simulink model "Distribution"  (R2018b)
settings: Solver=ode45  StartTime=0.0  StopTime=100  RelTol=1e-3
libraries: simeventslib x20
(part 1 of 2)
settings Model: Creator=tsprock3  LastModifiedBy=tas5
settings DataIOCC: LimitDataPoints=on  SaveFormat=Array
settings OptimizationCC: BlockReduction=off  BooleanDataType=off  LifeSpan=inf
settings DebuggingCC: SaveWithParameterizedLinksMsg=none  UnderspecifiedInitializationDetection=Classic  MergeDetectMultiDrivingBlocksExec=none  SignalResolutionControl=TryResolveAllWithWarning  AllowSymbolicDim=off  SFUnexpectedBacktrackingDiag=warning  SFNoUnconditionalDefaultTransitionDiag=warning  SFExecutionAtInitializationDiag=none
settings HardwareCC: ProdBitPerPointer=32  ProdBitPerSizeT=32  ProdBitPerPtrDiffT=32  ProdLargestAtomicFloat=None  ProdIntDivRoundTo=Undefined  ProdEndianess=Unspecified  ProdWordSize=32  ProdHWDeviceType=32-bit Generic  TargetUnknown=on
settings ModelReferenceCC: PropagateSignalLabelsOutOfModel=off
settings SFSimCC: SimUseLocalCustomCode=off
settings RTWCC: RTWUseLocalCustomCode=off
settings CodeAppCC: StateflowObjectComments=on
settings GRTTargetCC: TargetLangStandard=C89/C90 (ANSI)  GeneratePreprocessorConditionals=Disable all
settings ConfigComp: CovMetricSettings=dw  CovHtmlReporting=on  CovSaveCumulativeToWorkspaceVar=on  CovSaveSingleToWorkspaceVar=on  CovExternalEMLEnable=off
settings SimEventsCC: propMaxDesBlkSimulEvents=100000  propMaxDesMdlSimulEvents=1000000

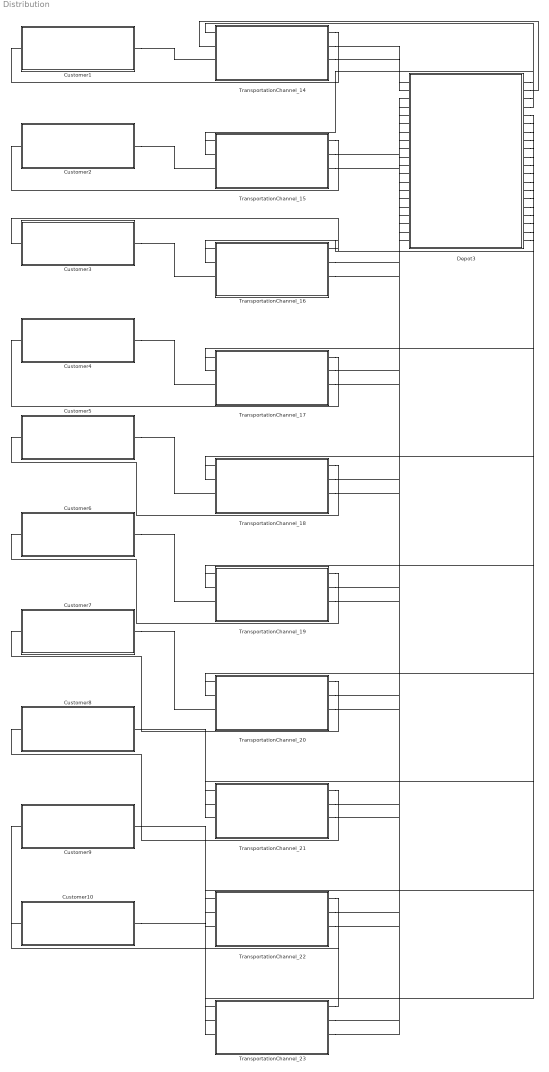
== system Distribution ==
  Customer1 : Subsystem
  Customer10 : Subsystem
  Customer2 : Subsystem
  Customer3 : Subsystem
  Customer4 : Subsystem
  Customer5 : Subsystem
  Customer6 : Subsystem
  Customer7 : Subsystem
  Customer8 : Subsystem
  Customer9 : Subsystem
  Depot3 : Subsystem
  TransportationChannel_14 : Subsystem
  TransportationChannel_15 : Subsystem
  TransportationChannel_16 : Subsystem
  TransportationChannel_17 : Subsystem
  TransportationChannel_18 : Subsystem
  TransportationChannel_19 : Subsystem
  TransportationChannel_20 : Subsystem
  TransportationChannel_21 : Subsystem
  TransportationChannel_22 : Subsystem
  TransportationChannel_23 : Subsystem
  connections:
  Depot3/RConn1 -- TransportationChannel_14/LConn1
  TransportationChannel_14/RConn1 -- Customer1/LConn1
  Depot3/RConn2 -- TransportationChannel_14/LConn2
  TransportationChannel_14/RConn2 -- Depot3/LConn1
  Customer1/RConn1 -- TransportationChannel_14/LConn3
  TransportationChannel_14/RConn3 -- Depot3/LConn2
  Depot3/RConn3 -- TransportationChannel_15/LConn1
  TransportationChannel_15/RConn1 -- Customer2/LConn1
  Depot3/RConn4 -- TransportationChannel_15/LConn2
  TransportationChannel_15/RConn2 -- Depot3/LConn3
  Customer2/RConn1 -- TransportationChannel_15/LConn3
  TransportationChannel_15/RConn3 -- Depot3/LConn4
  Depot3/RConn5 -- TransportationChannel_16/LConn1
  TransportationChannel_16/RConn1 -- Customer3/LConn1
  Depot3/RConn6 -- TransportationChannel_16/LConn2
  TransportationChannel_16/RConn2 -- Depot3/LConn5
  Customer3/RConn1 -- TransportationChannel_16/LConn3
  TransportationChannel_16/RConn3 -- Depot3/LConn6
  Depot3/RConn7 -- TransportationChannel_17/LConn1
  TransportationChannel_17/RConn1 -- Customer4/LConn1
  Depot3/RConn8 -- TransportationChannel_17/LConn2
  TransportationChannel_17/RConn2 -- Depot3/LConn7
  Customer4/RConn1 -- TransportationChannel_17/LConn3
  TransportationChannel_17/RConn3 -- Depot3/LConn8
  Depot3/RConn9 -- TransportationChannel_18/LConn1
  TransportationChannel_18/RConn1 -- Customer5/LConn1
  Depot3/RConn10 -- TransportationChannel_18/LConn2
  TransportationChannel_18/RConn2 -- Depot3/LConn9
  Customer5/RConn1 -- TransportationChannel_18/LConn3
  TransportationChannel_18/RConn3 -- Depot3/LConn10
  Depot3/RConn11 -- TransportationChannel_19/LConn1
  TransportationChannel_19/RConn1 -- Customer6/LConn1
  Depot3/RConn12 -- TransportationChannel_19/LConn2
  TransportationChannel_19/RConn2 -- Depot3/LConn11
  Customer6/RConn1 -- TransportationChannel_19/LConn3
  TransportationChannel_19/RConn3 -- Depot3/LConn12
  Depot3/RConn13 -- TransportationChannel_20/LConn1
  TransportationChannel_20/RConn1 -- Customer7/LConn1
  Depot3/RConn14 -- TransportationChannel_20/LConn2
  TransportationChannel_20/RConn2 -- Depot3/LConn13
  Customer7/RConn1 -- TransportationChannel_20/LConn3
  TransportationChannel_20/RConn3 -- Depot3/LConn14
  Depot3/RConn15 -- TransportationChannel_21/LConn1
  TransportationChannel_21/RConn1 -- Customer8/LConn1
  Depot3/RConn16 -- TransportationChannel_21/LConn2
  TransportationChannel_21/RConn2 -- Depot3/LConn15
  Customer8/RConn1 -- TransportationChannel_21/LConn3
  TransportationChannel_21/RConn3 -- Depot3/LConn16
  Depot3/RConn17 -- TransportationChannel_22/LConn1
  TransportationChannel_22/RConn1 -- Customer9/LConn1
  Depot3/RConn18 -- TransportationChannel_22/LConn2
  TransportationChannel_22/RConn2 -- Depot3/LConn17
  Customer9/RConn1 -- TransportationChannel_22/LConn3
  TransportationChannel_22/RConn3 -- Depot3/LConn18
  Depot3/RConn19 -- TransportationChannel_23/LConn1
  TransportationChannel_23/RConn1 -- Customer10/LConn1
  Depot3/RConn20 -- TransportationChannel_23/LConn2
  TransportationChannel_23/RConn2 -- Depot3/LConn19
  Customer10/RConn1 -- TransportationChannel_23/LConn3
  TransportationChannel_23/RConn3 -- Depot3/LConn20

== system Distribution/Customer1 ==
  AggregateCommodity : Subsystem  mask{Mean=2000/1459, AttributeValue=[1 0 1]|1|1|1}
      mask prompts: Mean "Frequency"; AttributeValue "Attributes"
      mask TypeOptions Mean: Source/Mean
      mask TypeOptions AttributeValue: setAttribute/AttributeValue
  Entity Sink : EntitySink
  Get Attribute : GetAttribute  AttributeName=Origin|Destination|Start  AttributeMissing=Error|Error|Error  AttributeDefaultValue=1|1|1  AttributeTreatAsVector=1|1|1  AttributeSendTiming=After entity departure|After entity departure|After entity departure  EvaluatedDefaultAttributeValue={[];[];[]}
      settings: OutputPortMap=o1,o2,o3
  IN_Commodity : PathCombiner  NumberInputPorts=1
  IN_Shipment : PathCombiner  NumberInputPorts=1
  Mux : Mux  Inputs=3
  OUT_Shipment : OutputSwitch  NumberOutputPorts=1  SwitchingCriterion=From signal port p  AttributeName=Customer  StatNumberDeparted=on
  Routing : EventBasedRandomNumber  Distribution=Arbitrary discrete  valueVecDisc=[0,1]  probVecDisc=[0,1]  Seed=57316
  Shipment_Metrics : simeventslib/SimEvents Sinks/Discrete Event Signal to Workspace  VariableName=Customer1  SaveFormat=Structure With Time  isMonitorOnly=off  isRecordIC=off
      settings: SourceProductName=SimEvents  SourceProductBaseCode=SE
  Signal Latch : SignalLatch  InitialMemoryValue=1  ReadMemoryUpon=Write to memory event
      settings: InputPortMap=u0,u2  OutputPortMap=o2
  inShipment_1 : PMIOPort  Side=Left
  outShipment_1 : PMIOPort  Port=2  Side=Right
  wires:
  Signal Latch/1 -> OUT_Shipment/1
  OUT_Shipment/1 -> Signal Latch/1
  Routing/1 -> Signal Latch/2
  Mux/1 -> Shipment_Metrics/1
  Get Attribute/3 -> Mux/3
  Get Attribute/2 -> Mux/2
  Get Attribute/1 -> Mux/1
  connections:
  IN_Commodity/RConn1 -- OUT_Shipment/LConn1
  Get Attribute/LConn1 -- IN_Shipment/RConn1
  Entity Sink/LConn1 -- Get Attribute/RConn1
  IN_Shipment/LConn1 -- inShipment_1/RConn1
  OUT_Shipment/RConn1 -- outShipment_1/RConn1
  AggregateCommodity/RConn1 -- IN_Commodity/LConn1

== system Distribution/Customer10 ==
  AggregateCommodity : Subsystem  mask{Mean=2000/2681, AttributeValue=[1 0 1]|1|1|1}
      mask prompts: Mean "Frequency"; AttributeValue "Attributes"
      mask TypeOptions Mean: Source/Mean
      mask TypeOptions AttributeValue: setAttribute/AttributeValue
  Entity Sink : EntitySink
  Get Attribute : GetAttribute  AttributeName=Origin|Destination|Start  AttributeMissing=Error|Error|Error  AttributeDefaultValue=1|1|1  AttributeTreatAsVector=1|1|1  AttributeSendTiming=After entity departure|After entity departure|After entity departure  EvaluatedDefaultAttributeValue={[];[];[]}
      settings: OutputPortMap=o1,o2,o3
  IN_Commodity : PathCombiner  NumberInputPorts=1
  IN_Shipment : PathCombiner  NumberInputPorts=1
  Mux : Mux  Inputs=3
  OUT_Shipment : OutputSwitch  NumberOutputPorts=1  SwitchingCriterion=From signal port p  AttributeName=Customer  StatNumberDeparted=on
  Routing : EventBasedRandomNumber  Distribution=Arbitrary discrete  valueVecDisc=[0,1]  probVecDisc=[0,1]  Seed=60533
  Shipment_Metrics : simeventslib/SimEvents Sinks/Discrete Event Signal to Workspace  VariableName=Customer10  SaveFormat=Structure With Time  isMonitorOnly=off  isRecordIC=off
      settings: SourceProductName=SimEvents  SourceProductBaseCode=SE
  Signal Latch : SignalLatch  InitialMemoryValue=1  ReadMemoryUpon=Write to memory event
      settings: InputPortMap=u0,u2  OutputPortMap=o2
  inShipment_1 : PMIOPort  Side=Left
  outShipment_1 : PMIOPort  Port=2  Side=Right
  wires:
  Signal Latch/1 -> OUT_Shipment/1
  OUT_Shipment/1 -> Signal Latch/1
  Routing/1 -> Signal Latch/2
  Mux/1 -> Shipment_Metrics/1
  Get Attribute/3 -> Mux/3
  Get Attribute/2 -> Mux/2
  Get Attribute/1 -> Mux/1
  connections:
  IN_Commodity/RConn1 -- OUT_Shipment/LConn1
  Get Attribute/LConn1 -- IN_Shipment/RConn1
  Entity Sink/LConn1 -- Get Attribute/RConn1
  IN_Shipment/LConn1 -- inShipment_1/RConn1
  OUT_Shipment/RConn1 -- outShipment_1/RConn1
  AggregateCommodity/RConn1 -- IN_Commodity/LConn1

== system Distribution/Customer2 ==
  AggregateCommodity : Subsystem  mask{Mean=2000/2296, AttributeValue=[1 0 1]|1|1|1}
      mask prompts: Mean "Frequency"; AttributeValue "Attributes"
      mask TypeOptions Mean: Source/Mean
      mask TypeOptions AttributeValue: setAttribute/AttributeValue
  Entity Sink : EntitySink
  Get Attribute : GetAttribute  AttributeName=Origin|Destination|Start  AttributeMissing=Error|Error|Error  AttributeDefaultValue=1|1|1  AttributeTreatAsVector=1|1|1  AttributeSendTiming=After entity departure|After entity departure|After entity departure  EvaluatedDefaultAttributeValue={[];[];[]}
      settings: OutputPortMap=o1,o2,o3
  IN_Commodity : PathCombiner  NumberInputPorts=1
  IN_Shipment : PathCombiner  NumberInputPorts=1
  Mux : Mux  Inputs=3
  OUT_Shipment : OutputSwitch  NumberOutputPorts=1  SwitchingCriterion=From signal port p  AttributeName=Customer  StatNumberDeparted=on
  Routing : EventBasedRandomNumber  Distribution=Arbitrary discrete  valueVecDisc=[0,1]  probVecDisc=[0,1]  Seed=63750
  Shipment_Metrics : simeventslib/SimEvents Sinks/Discrete Event Signal to Workspace  VariableName=Customer2  SaveFormat=Structure With Time  isMonitorOnly=off  isRecordIC=off
      settings: SourceProductName=SimEvents  SourceProductBaseCode=SE
  Signal Latch : SignalLatch  InitialMemoryValue=1  ReadMemoryUpon=Write to memory event
      settings: InputPortMap=u0,u2  OutputPortMap=o2
  inShipment_1 : PMIOPort  Side=Left
  outShipment_1 : PMIOPort  Port=2  Side=Right
  wires:
  Signal Latch/1 -> OUT_Shipment/1
  OUT_Shipment/1 -> Signal Latch/1
  Routing/1 -> Signal Latch/2
  Mux/1 -> Shipment_Metrics/1
  Get Attribute/3 -> Mux/3
  Get Attribute/2 -> Mux/2
  Get Attribute/1 -> Mux/1
  connections:
  IN_Commodity/RConn1 -- OUT_Shipment/LConn1
  Get Attribute/LConn1 -- IN_Shipment/RConn1
  Entity Sink/LConn1 -- Get Attribute/RConn1
  IN_Shipment/LConn1 -- inShipment_1/RConn1
  OUT_Shipment/RConn1 -- outShipment_1/RConn1
  AggregateCommodity/RConn1 -- IN_Commodity/LConn1

== system Distribution/Customer3 ==
  AggregateCommodity : Subsystem  mask{Mean=2000/1926, AttributeValue=[1 0 1]|1|1|1}
      mask prompts: Mean "Frequency"; AttributeValue "Attributes"
      mask TypeOptions Mean: Source/Mean
      mask TypeOptions AttributeValue: setAttribute/AttributeValue
  Entity Sink : EntitySink
  Get Attribute : GetAttribute  AttributeName=Origin|Destination|Start  AttributeMissing=Error|Error|Error  AttributeDefaultValue=1|1|1  AttributeTreatAsVector=1|1|1  AttributeSendTiming=After entity departure|After entity departure|After entity departure  EvaluatedDefaultAttributeValue={[];[];[]}
      settings: OutputPortMap=o1,o2,o3
  IN_Commodity : PathCombiner  NumberInputPorts=1
  IN_Shipment : PathCombiner  NumberInputPorts=1
  Mux : Mux  Inputs=3
  OUT_Shipment : OutputSwitch  NumberOutputPorts=1  SwitchingCriterion=From signal port p  AttributeName=Customer  StatNumberDeparted=on
  Routing : EventBasedRandomNumber  Distribution=Arbitrary discrete  valueVecDisc=[0,1]  probVecDisc=[0,1]  Seed=1431
  Shipment_Metrics : simeventslib/SimEvents Sinks/Discrete Event Signal to Workspace  VariableName=Customer3  SaveFormat=Structure With Time  isMonitorOnly=off  isRecordIC=off
      settings: SourceProductName=SimEvents  SourceProductBaseCode=SE
  Signal Latch : SignalLatch  InitialMemoryValue=1  ReadMemoryUpon=Write to memory event
      settings: InputPortMap=u0,u2  OutputPortMap=o2
  inShipment_1 : PMIOPort  Side=Left
  outShipment_1 : PMIOPort  Port=2  Side=Right
  wires:
  Signal Latch/1 -> OUT_Shipment/1
  OUT_Shipment/1 -> Signal Latch/1
  Routing/1 -> Signal Latch/2
  Mux/1 -> Shipment_Metrics/1
  Get Attribute/3 -> Mux/3
  Get Attribute/2 -> Mux/2
  Get Attribute/1 -> Mux/1
  connections:
  IN_Commodity/RConn1 -- OUT_Shipment/LConn1
  Get Attribute/LConn1 -- IN_Shipment/RConn1
  Entity Sink/LConn1 -- Get Attribute/RConn1
  IN_Shipment/LConn1 -- inShipment_1/RConn1
  OUT_Shipment/RConn1 -- outShipment_1/RConn1
  AggregateCommodity/RConn1 -- IN_Commodity/LConn1

== system Distribution/Customer4 ==
  AggregateCommodity : Subsystem  mask{Mean=2000/1531, AttributeValue=[1 0 1]|1|1|1}
      mask prompts: Mean "Frequency"; AttributeValue "Attributes"
      mask TypeOptions Mean: Source/Mean
      mask TypeOptions AttributeValue: setAttribute/AttributeValue
  Entity Sink : EntitySink
  Get Attribute : GetAttribute  AttributeName=Origin|Destination|Start  AttributeMissing=Error|Error|Error  AttributeDefaultValue=1|1|1  AttributeTreatAsVector=1|1|1  AttributeSendTiming=After entity departure|After entity departure|After entity departure  EvaluatedDefaultAttributeValue={[];[];[]}
      settings: OutputPortMap=o1,o2,o3
  IN_Commodity : PathCombiner  NumberInputPorts=1
  IN_Shipment : PathCombiner  NumberInputPorts=1
  Mux : Mux  Inputs=3
  OUT_Shipment : OutputSwitch  NumberOutputPorts=1  SwitchingCriterion=From signal port p  AttributeName=Customer  StatNumberDeparted=on
  Routing : EventBasedRandomNumber  Distribution=Arbitrary discrete  valueVecDisc=[0,1]  probVecDisc=[0,1]  Seed=4648
  Shipment_Metrics : simeventslib/SimEvents Sinks/Discrete Event Signal to Workspace  VariableName=Customer4  SaveFormat=Structure With Time  isMonitorOnly=off  isRecordIC=off
      settings: SourceProductName=SimEvents  SourceProductBaseCode=SE
  Signal Latch : SignalLatch  InitialMemoryValue=1  ReadMemoryUpon=Write to memory event
      settings: InputPortMap=u0,u2  OutputPortMap=o2
  inShipment_1 : PMIOPort  Side=Left
  outShipment_1 : PMIOPort  Port=2  Side=Right
  wires:
  Signal Latch/1 -> OUT_Shipment/1
  OUT_Shipment/1 -> Signal Latch/1
  Routing/1 -> Signal Latch/2
  Mux/1 -> Shipment_Metrics/1
  Get Attribute/3 -> Mux/3
  Get Attribute/2 -> Mux/2
  Get Attribute/1 -> Mux/1
  connections:
  IN_Commodity/RConn1 -- OUT_Shipment/LConn1
  Get Attribute/LConn1 -- IN_Shipment/RConn1
  Entity Sink/LConn1 -- Get Attribute/RConn1
  IN_Shipment/LConn1 -- inShipment_1/RConn1
  OUT_Shipment/RConn1 -- outShipment_1/RConn1
  AggregateCommodity/RConn1 -- IN_Commodity/LConn1

== system Distribution/Customer5 ==
  AggregateCommodity : Subsystem  mask{Mean=2000/1642, AttributeValue=[1 0 1]|1|1|1}
      mask prompts: Mean "Frequency"; AttributeValue "Attributes"
      mask TypeOptions Mean: Source/Mean
      mask TypeOptions AttributeValue: setAttribute/AttributeValue
  Entity Sink : EntitySink
  Get Attribute : GetAttribute  AttributeName=Origin|Destination|Start  AttributeMissing=Error|Error|Error  AttributeDefaultValue=1|1|1  AttributeTreatAsVector=1|1|1  AttributeSendTiming=After entity departure|After entity departure|After entity departure  EvaluatedDefaultAttributeValue={[];[];[]}
      settings: OutputPortMap=o1,o2,o3
  IN_Commodity : PathCombiner  NumberInputPorts=1
  IN_Shipment : PathCombiner  NumberInputPorts=1
  Mux : Mux  Inputs=3
  OUT_Shipment : OutputSwitch  NumberOutputPorts=1  SwitchingCriterion=From signal port p  AttributeName=Customer  StatNumberDeparted=on
  Routing : EventBasedRandomNumber  Distribution=Arbitrary discrete  valueVecDisc=[0,1]  probVecDisc=[0,1]  Seed=7865
  Shipment_Metrics : simeventslib/SimEvents Sinks/Discrete Event Signal to Workspace  VariableName=Customer5  SaveFormat=Structure With Time  isMonitorOnly=off  isRecordIC=off
      settings: SourceProductName=SimEvents  SourceProductBaseCode=SE
  Signal Latch : SignalLatch  InitialMemoryValue=1  ReadMemoryUpon=Write to memory event
      settings: InputPortMap=u0,u2  OutputPortMap=o2
  inShipment_1 : PMIOPort  Side=Left
  outShipment_1 : PMIOPort  Port=2  Side=Right
  wires:
  Signal Latch/1 -> OUT_Shipment/1
  OUT_Shipment/1 -> Signal Latch/1
  Routing/1 -> Signal Latch/2
  Mux/1 -> Shipment_Metrics/1
  Get Attribute/3 -> Mux/3
  Get Attribute/2 -> Mux/2
  Get Attribute/1 -> Mux/1
  connections:
  IN_Commodity/RConn1 -- OUT_Shipment/LConn1
  Get Attribute/LConn1 -- IN_Shipment/RConn1
  Entity Sink/LConn1 -- Get Attribute/RConn1
  IN_Shipment/LConn1 -- inShipment_1/RConn1
  OUT_Shipment/RConn1 -- outShipment_1/RConn1
  AggregateCommodity/RConn1 -- IN_Commodity/LConn1

== system Distribution/Customer6 ==
  AggregateCommodity : Subsystem  mask{Mean=2000/2502, AttributeValue=[1 0 1]|1|1|1}
      mask prompts: Mean "Frequency"; AttributeValue "Attributes"
      mask TypeOptions Mean: Source/Mean
      mask TypeOptions AttributeValue: setAttribute/AttributeValue
  Entity Sink : EntitySink
  Get Attribute : GetAttribute  AttributeName=Origin|Destination|Start  AttributeMissing=Error|Error|Error  AttributeDefaultValue=1|1|1  AttributeTreatAsVector=1|1|1  AttributeSendTiming=After entity departure|After entity departure|After entity departure  EvaluatedDefaultAttributeValue={[];[];[]}
      settings: OutputPortMap=o1,o2,o3
  IN_Commodity : PathCombiner  NumberInputPorts=1
  IN_Shipment : PathCombiner  NumberInputPorts=1
  Mux : Mux  Inputs=3
  OUT_Shipment : OutputSwitch  NumberOutputPorts=1  SwitchingCriterion=From signal port p  AttributeName=Customer  StatNumberDeparted=on
  Routing : EventBasedRandomNumber  Distribution=Arbitrary discrete  valueVecDisc=[0,1]  probVecDisc=[0,1]  Seed=11082
  Shipment_Metrics : simeventslib/SimEvents Sinks/Discrete Event Signal to Workspace  VariableName=Customer6  SaveFormat=Structure With Time  isMonitorOnly=off  isRecordIC=off
      settings: SourceProductName=SimEvents  SourceProductBaseCode=SE
  Signal Latch : SignalLatch  InitialMemoryValue=1  ReadMemoryUpon=Write to memory event
      settings: InputPortMap=u0,u2  OutputPortMap=o2
  inShipment_1 : PMIOPort  Side=Left
  outShipment_1 : PMIOPort  Port=2  Side=Right
  wires:
  Signal Latch/1 -> OUT_Shipment/1
  OUT_Shipment/1 -> Signal Latch/1
  Routing/1 -> Signal Latch/2
  Mux/1 -> Shipment_Metrics/1
  Get Attribute/3 -> Mux/3
  Get Attribute/2 -> Mux/2
  Get Attribute/1 -> Mux/1
  connections:
  IN_Commodity/RConn1 -- OUT_Shipment/LConn1
  Get Attribute/LConn1 -- IN_Shipment/RConn1
  Entity Sink/LConn1 -- Get Attribute/RConn1
  IN_Shipment/LConn1 -- inShipment_1/RConn1
  OUT_Shipment/RConn1 -- outShipment_1/RConn1
  AggregateCommodity/RConn1 -- IN_Commodity/LConn1

== system Distribution/Customer7 ==
  AggregateCommodity : Subsystem  mask{Mean=2000/2136, AttributeValue=[1 0 1]|1|1|1}
      mask prompts: Mean "Frequency"; AttributeValue "Attributes"
      mask TypeOptions Mean: Source/Mean
      mask TypeOptions AttributeValue: setAttribute/AttributeValue
  Entity Sink : EntitySink
  Get Attribute : GetAttribute  AttributeName=Origin|Destination|Start  AttributeMissing=Error|Error|Error  AttributeDefaultValue=1|1|1  AttributeTreatAsVector=1|1|1  AttributeSendTiming=After entity departure|After entity departure|After entity departure  EvaluatedDefaultAttributeValue={[];[];[]}
      settings: OutputPortMap=o1,o2,o3
  IN_Commodity : PathCombiner  NumberInputPorts=1
  IN_Shipment : PathCombiner  NumberInputPorts=1
  Mux : Mux  Inputs=3
  OUT_Shipment : OutputSwitch  NumberOutputPorts=1  SwitchingCriterion=From signal port p  AttributeName=Customer  StatNumberDeparted=on
  Routing : EventBasedRandomNumber  Distribution=Arbitrary discrete  valueVecDisc=[0,1]  probVecDisc=[0,1]  Seed=14299
  Shipment_Metrics : simeventslib/SimEvents Sinks/Discrete Event Signal to Workspace  VariableName=Customer7  SaveFormat=Structure With Time  isMonitorOnly=off  isRecordIC=off
      settings: SourceProductName=SimEvents  SourceProductBaseCode=SE
  Signal Latch : SignalLatch  InitialMemoryValue=1  ReadMemoryUpon=Write to memory event
      settings: InputPortMap=u0,u2  OutputPortMap=o2
  inShipment_1 : PMIOPort  Side=Left
  outShipment_1 : PMIOPort  Port=2  Side=Right
  wires:
  Signal Latch/1 -> OUT_Shipment/1
  OUT_Shipment/1 -> Signal Latch/1
  Routing/1 -> Signal Latch/2
  Mux/1 -> Shipment_Metrics/1
  Get Attribute/3 -> Mux/3
  Get Attribute/2 -> Mux/2
  Get Attribute/1 -> Mux/1
  connections:
  IN_Commodity/RConn1 -- OUT_Shipment/LConn1
  Get Attribute/LConn1 -- IN_Shipment/RConn1
  Entity Sink/LConn1 -- Get Attribute/RConn1
  IN_Shipment/LConn1 -- inShipment_1/RConn1
  OUT_Shipment/RConn1 -- outShipment_1/RConn1
  AggregateCommodity/RConn1 -- IN_Commodity/LConn1

== system Distribution/Customer8 ==
  AggregateCommodity : Subsystem  mask{Mean=2000/1826, AttributeValue=[1 0 1]|1|1|1}
      mask prompts: Mean "Frequency"; AttributeValue "Attributes"
      mask TypeOptions Mean: Source/Mean
      mask TypeOptions AttributeValue: setAttribute/AttributeValue
  Entity Sink : EntitySink
  Get Attribute : GetAttribute  AttributeName=Origin|Destination|Start  AttributeMissing=Error|Error|Error  AttributeDefaultValue=1|1|1  AttributeTreatAsVector=1|1|1  AttributeSendTiming=After entity departure|After entity departure|After entity departure  EvaluatedDefaultAttributeValue={[];[];[]}
      settings: OutputPortMap=o1,o2,o3
  IN_Commodity : PathCombiner  NumberInputPorts=1
  IN_Shipment : PathCombiner  NumberInputPorts=1
  Mux : Mux  Inputs=3
  OUT_Shipment : OutputSwitch  NumberOutputPorts=1  SwitchingCriterion=From signal port p  AttributeName=Customer  StatNumberDeparted=on
  Routing : EventBasedRandomNumber  Distribution=Arbitrary discrete  valueVecDisc=[0,1]  probVecDisc=[0,1]  Seed=17516
  Shipment_Metrics : simeventslib/SimEvents Sinks/Discrete Event Signal to Workspace  VariableName=Customer8  SaveFormat=Structure With Time  isMonitorOnly=off  isRecordIC=off
      settings: SourceProductName=SimEvents  SourceProductBaseCode=SE
  Signal Latch : SignalLatch  InitialMemoryValue=1  ReadMemoryUpon=Write to memory event
      settings: InputPortMap=u0,u2  OutputPortMap=o2
  inShipment_1 : PMIOPort  Side=Left
  outShipment_1 : PMIOPort  Port=2  Side=Right
  wires:
  Signal Latch/1 -> OUT_Shipment/1
  OUT_Shipment/1 -> Signal Latch/1
  Routing/1 -> Signal Latch/2
  Mux/1 -> Shipment_Metrics/1
  Get Attribute/3 -> Mux/3
  Get Attribute/2 -> Mux/2
  Get Attribute/1 -> Mux/1
  connections:
  IN_Commodity/RConn1 -- OUT_Shipment/LConn1
  Get Attribute/LConn1 -- IN_Shipment/RConn1
  Entity Sink/LConn1 -- Get Attribute/RConn1
  IN_Shipment/LConn1 -- inShipment_1/RConn1
  OUT_Shipment/RConn1 -- outShipment_1/RConn1
  AggregateCommodity/RConn1 -- IN_Commodity/LConn1

== system Distribution/Customer9 ==
  AggregateCommodity : Subsystem  mask{Mean=2000/871, AttributeValue=[1 0 1]|1|1|1}
      mask prompts: Mean "Frequency"; AttributeValue "Attributes"
      mask TypeOptions Mean: Source/Mean
      mask TypeOptions AttributeValue: setAttribute/AttributeValue
  Entity Sink : EntitySink
  Get Attribute : GetAttribute  AttributeName=Origin|Destination|Start  AttributeMissing=Error|Error|Error  AttributeDefaultValue=1|1|1  AttributeTreatAsVector=1|1|1  AttributeSendTiming=After entity departure|After entity departure|After entity departure  EvaluatedDefaultAttributeValue={[];[];[]}
      settings: OutputPortMap=o1,o2,o3
  IN_Commodity : PathCombiner  NumberInputPorts=1
  IN_Shipment : PathCombiner  NumberInputPorts=1
  Mux : Mux  Inputs=3
  OUT_Shipment : OutputSwitch  NumberOutputPorts=1  SwitchingCriterion=From signal port p  AttributeName=Customer  StatNumberDeparted=on
  Routing : EventBasedRandomNumber  Distribution=Arbitrary discrete  valueVecDisc=[0,1]  probVecDisc=[0,1]  Seed=20733
  Shipment_Metrics : simeventslib/SimEvents Sinks/Discrete Event Signal to Workspace  VariableName=Customer9  SaveFormat=Structure With Time  isMonitorOnly=off  isRecordIC=off
      settings: SourceProductName=SimEvents  SourceProductBaseCode=SE
  Signal Latch : SignalLatch  InitialMemoryValue=1  ReadMemoryUpon=Write to memory event
      settings: InputPortMap=u0,u2  OutputPortMap=o2
  inShipment_1 : PMIOPort  Side=Left
  outShipment_1 : PMIOPort  Port=2  Side=Right
  wires:
  Signal Latch/1 -> OUT_Shipment/1
  OUT_Shipment/1 -> Signal Latch/1
  Routing/1 -> Signal Latch/2
  Mux/1 -> Shipment_Metrics/1
  Get Attribute/3 -> Mux/3
  Get Attribute/2 -> Mux/2
  Get Attribute/1 -> Mux/1
  connections:
  IN_Commodity/RConn1 -- OUT_Shipment/LConn1
  Get Attribute/LConn1 -- IN_Shipment/RConn1
  Entity Sink/LConn1 -- Get Attribute/RConn1
  IN_Shipment/LConn1 -- inShipment_1/RConn1
  OUT_Shipment/RConn1 -- outShipment_1/RConn1
  AggregateCommodity/RConn1 -- IN_Commodity/LConn1

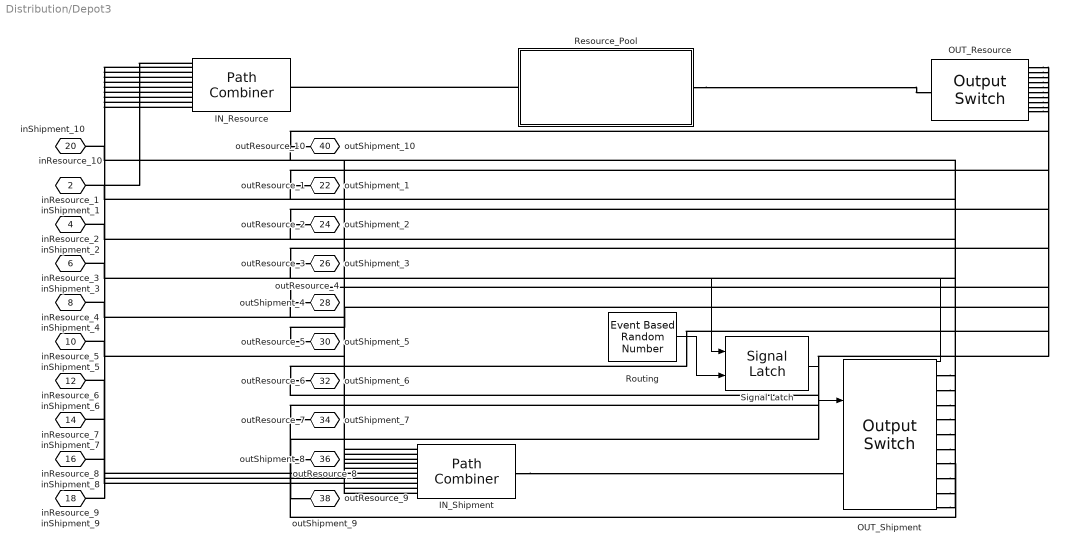
== system Distribution/Depot3 ==
  IN_Resource : PathCombiner  NumberInputPorts=10
  IN_Shipment : PathCombiner  NumberInputPorts=10
  OUT_Resource : OutputSwitch  NumberOutputPorts=10  SwitchingCriterion=Round robin  InitialSeed=57769
  OUT_Shipment : OutputSwitch  NumberOutputPorts=10  SwitchingCriterion=From signal port p  AttributeName=Customer  StatNumberDeparted=on
  Resource_Pool : Subsystem  mask{Quantity=6}
      mask prompts: Quantity "How many entities in resource pool?"
      mask TypeOptions Quantity:
      | Time-Based
      | Function-Call Generator/NumberOfEventsPerPeriod
  Routing : EventBasedRandomNumber  Distribution=Arbitrary discrete  valueVecDisc=[0,1,2,3,4,5,6,7,8,9,10]  probVecDisc=[0,0.0908,0.0914,0.1042,0.1372,0.0772,0.0447,0.1159,0.1513,0.0905,0.0968]  Seed=23950
  Signal Latch : SignalLatch  InitialMemoryValue=1  ReadMemoryUpon=Write to memory event
      settings: InputPortMap=u0,u2  OutputPortMap=o2
  inResource_1 : PMIOPort  Side=Left
  inShipment_1 : PMIOPort  Port=2  Side=Left
  inResource_2 : PMIOPort  Port=3  Side=Left
  inShipment_2 : PMIOPort  Port=4  Side=Left
  inResource_3 : PMIOPort  Port=5  Side=Left
  inShipment_3 : PMIOPort  Port=6  Side=Left
  inResource_4 : PMIOPort  Port=7  Side=Left
  inShipment_4 : PMIOPort  Port=8  Side=Left
  inResource_5 : PMIOPort  Port=9  Side=Left
  inShipment_5 : PMIOPort  Port=10  Side=Left
  inResource_6 : PMIOPort  Port=11  Side=Left
  inShipment_6 : PMIOPort  Port=12  Side=Left
  inResource_7 : PMIOPort  Port=13  Side=Left
  inShipment_7 : PMIOPort  Port=14  Side=Left
  inResource_8 : PMIOPort  Port=15  Side=Left
  inShipment_8 : PMIOPort  Port=16  Side=Left
  inResource_9 : PMIOPort  Port=17  Side=Left
  inShipment_9 : PMIOPort  Port=18  Side=Left
  inResource_10 : PMIOPort  Port=19  Side=Left
  inShipment_10 : PMIOPort  Port=20  Side=Left
  outShipment_1 : PMIOPort  Port=21  Side=Right
  outResource_1 : PMIOPort  Port=22  Side=Right
  outShipment_2 : PMIOPort  Port=23  Side=Right
  outResource_2 : PMIOPort  Port=24  Side=Right
  outShipment_3 : PMIOPort  Port=25  Side=Right
  outResource_3 : PMIOPort  Port=26  Side=Right
  outShipment_4 : PMIOPort  Port=27  Side=Right
  outResource_4 : PMIOPort  Port=28  Side=Right
  outShipment_5 : PMIOPort  Port=29  Side=Right
  outResource_5 : PMIOPort  Port=30  Side=Right
  outShipment_6 : PMIOPort  Port=31  Side=Right
  outResource_6 : PMIOPort  Port=32  Side=Right
  outShipment_7 : PMIOPort  Port=33  Side=Right
  outResource_7 : PMIOPort  Port=34  Side=Right
  outShipment_8 : PMIOPort  Port=35  Side=Right
  outResource_8 : PMIOPort  Port=36  Side=Right
  outShipment_9 : PMIOPort  Port=37  Side=Right
  outResource_9 : PMIOPort  Port=38  Side=Right
  outShipment_10 : PMIOPort  Port=39  Side=Right
  outResource_10 : PMIOPort  Port=40  Side=Right
  wires:
  OUT_Shipment/1 -> Signal Latch/1
  Routing/1 -> Signal Latch/2
  Signal Latch/1 -> OUT_Shipment/1
  connections:
  Resource_Pool/LConn1 -- OUT_Resource/LConn1
  IN_Shipment/RConn1 -- OUT_Shipment/LConn1
  Resource_Pool/RConn1 -- IN_Resource/RConn1
  IN_Resource/LConn1 -- inResource_1/RConn1
  IN_Resource/LConn2 -- inResource_2/RConn1
  IN_Resource/LConn3 -- inResource_3/RConn1
  IN_Resource/LConn4 -- inResource_4/RConn1
  IN_Resource/LConn5 -- inResource_5/RConn1
  IN_Resource/LConn6 -- inResource_6/RConn1
  IN_Resource/LConn7 -- inResource_7/RConn1
  IN_Resource/LConn8 -- inResource_8/RConn1
  IN_Resource/LConn9 -- inResource_9/RConn1
  IN_Resource/LConn10 -- inResource_10/RConn1
  OUT_Resource/RConn1 -- outResource_1/RConn1
  OUT_Resource/RConn2 -- outResource_2/RConn1
  OUT_Resource/RConn3 -- outResource_3/RConn1
  OUT_Resource/RConn4 -- outResource_4/RConn1
  OUT_Resource/RConn5 -- outResource_5/RConn1
  OUT_Resource/RConn6 -- outResource_6/RConn1
  OUT_Resource/RConn7 -- outResource_7/RConn1
  OUT_Resource/RConn8 -- outResource_8/RConn1
  OUT_Resource/RConn9 -- outResource_9/RConn1
  OUT_Resource/RConn10 -- outResource_10/RConn1
  IN_Shipment/LConn1 -- inShipment_1/RConn1
  IN_Shipment/LConn2 -- inShipment_2/RConn1
  IN_Shipment/LConn3 -- inShipment_3/RConn1
  IN_Shipment/LConn4 -- inShipment_4/RConn1
  IN_Shipment/LConn5 -- inShipment_5/RConn1
  IN_Shipment/LConn6 -- inShipment_6/RConn1
  IN_Shipment/LConn7 -- inShipment_7/RConn1
  IN_Shipment/LConn8 -- inShipment_8/RConn1
  IN_Shipment/LConn9 -- inShipment_9/RConn1
  IN_Shipment/LConn10 -- inShipment_10/RConn1
  OUT_Shipment/RConn1 -- outShipment_1/RConn1
  OUT_Shipment/RConn2 -- outShipment_2/RConn1
  OUT_Shipment/RConn3 -- outShipment_3/RConn1
  OUT_Shipment/RConn4 -- outShipment_4/RConn1
  OUT_Shipment/RConn5 -- outShipment_5/RConn1
  OUT_Shipment/RConn6 -- outShipment_6/RConn1
  OUT_Shipment/RConn7 -- outShipment_7/RConn1
  OUT_Shipment/RConn8 -- outShipment_8/RConn1
  OUT_Shipment/RConn9 -- outShipment_9/RConn1
  OUT_Shipment/RConn10 -- outShipment_10/RConn1

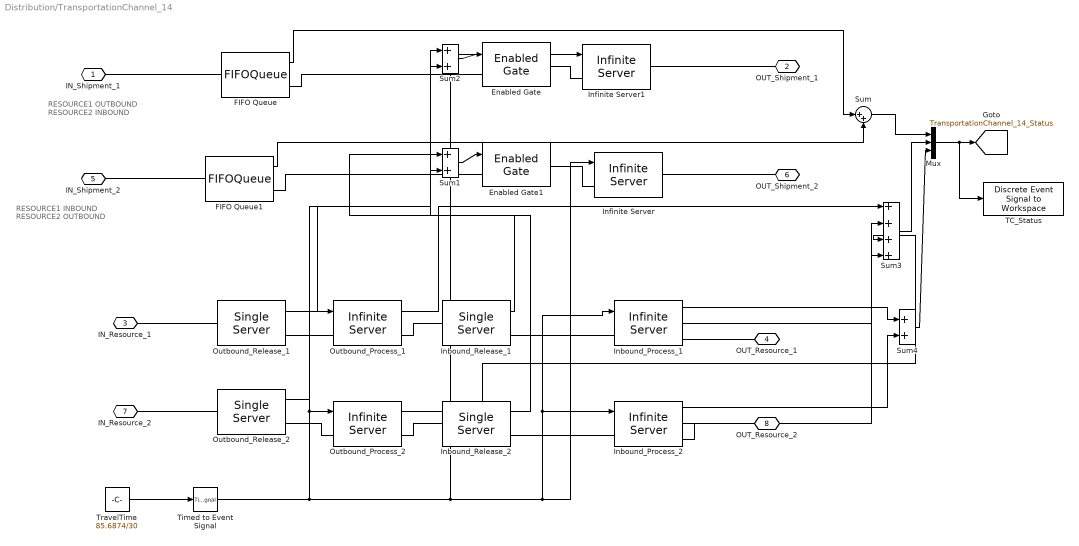
== system Distribution/TransportationChannel_14 ==
  note: RESOURCE1 OUTBOUND
      | RESOURCE2 INBOUND
  note: RESOURCE1 INBOUND
      | RESOURCE2 OUTBOUND
  Enabled Gate : EnabledGate
  Enabled Gate1 : EnabledGate
  FIFO Queue : FIFOQueue  Capacity=inf  StatNumberInBlock=on
      settings: OutputPortMap=o1
  FIFO Queue1 : FIFOQueue  Capacity=inf  StatNumberInBlock=on
      settings: OutputPortMap=o1
  Inbound_Process_1 : InfiniteServer  ServiceTimeFrom=Signal port t  ServiceTime=(76.7)/30  StatNumberDeparted=on  StatNumberInBlock=on
      settings: OutputPortMap=o0,o1
  Inbound_Process_2 : InfiniteServer  ServiceTimeFrom=Signal port t  ServiceTime=(76.7)/30  StatNumberDeparted=on  StatNumberInBlock=on
      settings: OutputPortMap=o0,o1
  Inbound_Release_1 : SingleServer  ServiceTime=0  StatNumberInBlock=on
      settings: OutputPortMap=o1
  Inbound_Release_2 : SingleServer  ServiceTime=0  StatNumberInBlock=on
      settings: OutputPortMap=o1
  Infinite Server : InfiniteServer  ServiceTimeFrom=Signal port t  ServiceTime=(76.7)/30
  Infinite Server1 : InfiniteServer  ServiceTimeFrom=Signal port t  ServiceTime=(76.7)/30
  Mux : Mux  Inputs=3
  Outbound_Process_1 : InfiniteServer  ServiceTimeFrom=Signal port t  ServiceTime=(76.7)/30  StatNumberInBlock=on
      settings: OutputPortMap=o1
  Outbound_Process_2 : InfiniteServer  ServiceTimeFrom=Signal port t  ServiceTime=(76.7)/30  StatNumberInBlock=on
      settings: OutputPortMap=o1
  Outbound_Release_1 : SingleServer  ServiceTime=0  StatNumberInBlock=on
      settings: OutputPortMap=o1
  Outbound_Release_2 : SingleServer  ServiceTime=0  StatNumberInBlock=on
      settings: OutputPortMap=o1
  Sum{,1..2,4} (4 alike) : Sum  Inputs=|++
  Sum3 : Sum  Inputs=|++++
  TC_Status : simeventslib/SimEvents Sinks/Discrete Event Signal to Workspace  VariableName=TransportationChannel_14_Status  SaveFormat=Structure With Time  isMonitorOnly=off  isRecordIC=off
      settings: SourceProductName=SimEvents  SourceProductBaseCode=SE
  Timed to Event Signal : TimedToEventSignal
  TravelTime : Constant  Value=85.6874/30
  IN_Shipment_1 : PMIOPort  Side=Left
  OUT_Shipment_1 : PMIOPort  Port=2  Side=Right
  IN_Resource_1 : PMIOPort  Port=3  Side=Left
  OUT_Resource_1 : PMIOPort  Port=4  Side=Right
  IN_Shipment_2 : PMIOPort  Port=5  Side=Left
  OUT_Shipment_2 : PMIOPort  Port=6  Side=Right
  IN_Resource_2 : PMIOPort  Port=7  Side=Left
  OUT_Resource_2 : PMIOPort  Port=8  Side=Right
  tag scope: TransportationChannel_14_Status=global
  wires:
  Sum4/1 -> Mux/3
  Inbound_Process_2/1 -> Sum4/2
  Inbound_Process_1/1 -> Sum4/1
  Inbound_Process_2/2 -> Sum3/4
  Outbound_Process_2/1 -> Sum3/3
  Inbound_Process_1/2 -> Sum3/2
  Outbound_Process_1/1 -> Sum3/1
  Sum3/1 -> Mux/2
  Sum/1 -> Mux/1
  Mux/1 -> TC_Status/1, [TransportationChannel_14_Status]
  Inbound_Release_2/1 -> Sum2/2
  Outbound_Release_1/1 -> Sum2/1
  Sum2/1 -> Enabled Gate/1
  Inbound_Release_1/1 -> Sum1/1
  Outbound_Release_2/1 -> Sum1/2
  Sum1/1 -> Enabled Gate1/1
  Timed to Event Signal/1 -> Outbound_Process_2/1, Outbound_Process_1/1, Infinite Server1/1, Inbound_Process_2/1, Inbound_Process_1/1, Infinite Server/1
  TravelTime/1 -> Timed to Event Signal/1
  FIFO Queue/1 -> Sum/1
  FIFO Queue1/1 -> Sum/2
  connections:
  Inbound_Process_1/RConn1 -- OUT_Resource_1/RConn1
  Outbound_Process_1/RConn1 -- Inbound_Release_1/LConn1
  Inbound_Release_1/RConn1 -- Inbound_Process_1/LConn1
  Outbound_Release_1/RConn1 -- Outbound_Process_1/LConn1
  Inbound_Process_2/RConn1 -- OUT_Resource_2/RConn1
  Inbound_Release_2/RConn1 -- Inbound_Process_2/LConn1
  Outbound_Process_2/RConn1 -- Inbound_Release_2/LConn1
  Outbound_Release_2/RConn1 -- Outbound_Process_2/LConn1
  IN_Resource_2/RConn1 -- Outbound_Release_2/LConn1
  Infinite Server1/RConn1 -- OUT_Shipment_1/RConn1
  Enabled Gate/RConn1 -- Infinite Server1/LConn1
  Infinite Server/LConn1 -- Enabled Gate1/RConn1
  OUT_Shipment_2/RConn1 -- Infinite Server/RConn1
  IN_Resource_1/RConn1 -- Outbound_Release_1/LConn1
  IN_Shipment_2/RConn1 -- FIFO Queue1/LConn1
  IN_Shipment_1/RConn1 -- FIFO Queue/LConn1
  Enabled Gate1/LConn1 -- FIFO Queue1/RConn1
  FIFO Queue/RConn1 -- Enabled Gate/LConn1

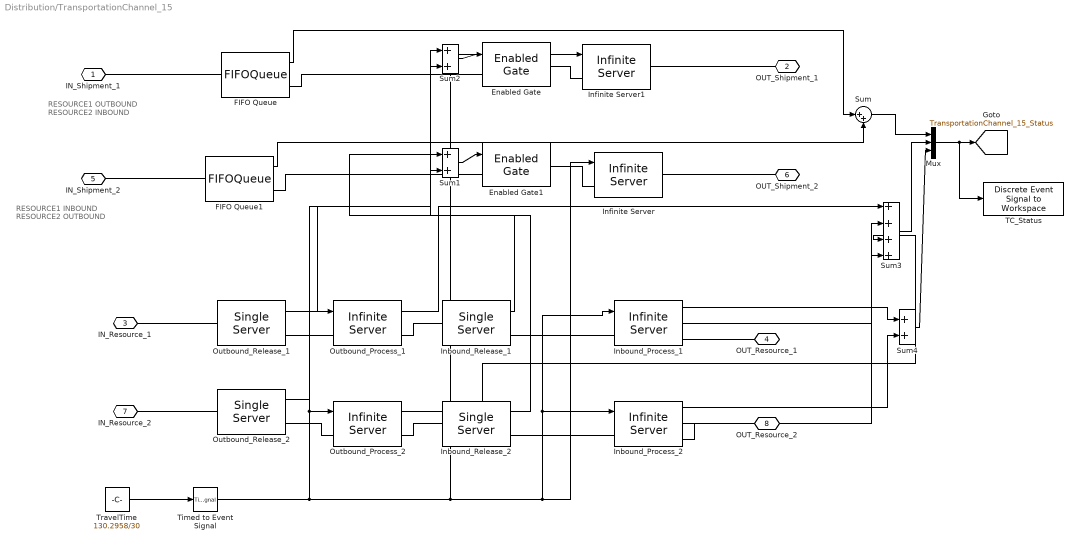
== system Distribution/TransportationChannel_15 ==
  note: RESOURCE1 OUTBOUND
      | RESOURCE2 INBOUND
  note: RESOURCE1 INBOUND
      | RESOURCE2 OUTBOUND
  Enabled Gate : EnabledGate
  Enabled Gate1 : EnabledGate
  FIFO Queue : FIFOQueue  Capacity=inf  StatNumberInBlock=on
      settings: OutputPortMap=o1
  FIFO Queue1 : FIFOQueue  Capacity=inf  StatNumberInBlock=on
      settings: OutputPortMap=o1
  Inbound_Process_1 : InfiniteServer  ServiceTimeFrom=Signal port t  ServiceTime=(76.7)/30  StatNumberDeparted=on  StatNumberInBlock=on
      settings: OutputPortMap=o0,o1
  Inbound_Process_2 : InfiniteServer  ServiceTimeFrom=Signal port t  ServiceTime=(76.7)/30  StatNumberDeparted=on  StatNumberInBlock=on
      settings: OutputPortMap=o0,o1
  Inbound_Release_1 : SingleServer  ServiceTime=0  StatNumberInBlock=on
      settings: OutputPortMap=o1
  Inbound_Release_2 : SingleServer  ServiceTime=0  StatNumberInBlock=on
      settings: OutputPortMap=o1
  Infinite Server : InfiniteServer  ServiceTimeFrom=Signal port t  ServiceTime=(76.7)/30
  Infinite Server1 : InfiniteServer  ServiceTimeFrom=Signal port t  ServiceTime=(76.7)/30
  Mux : Mux  Inputs=3
  Outbound_Process_1 : InfiniteServer  ServiceTimeFrom=Signal port t  ServiceTime=(76.7)/30  StatNumberInBlock=on
      settings: OutputPortMap=o1
  Outbound_Process_2 : InfiniteServer  ServiceTimeFrom=Signal port t  ServiceTime=(76.7)/30  StatNumberInBlock=on
      settings: OutputPortMap=o1
  Outbound_Release_1 : SingleServer  ServiceTime=0  StatNumberInBlock=on
      settings: OutputPortMap=o1
  Outbound_Release_2 : SingleServer  ServiceTime=0  StatNumberInBlock=on
      settings: OutputPortMap=o1
  Sum{,1..2,4} (4 alike) : Sum  Inputs=|++
  Sum3 : Sum  Inputs=|++++
  TC_Status : simeventslib/SimEvents Sinks/Discrete Event Signal to Workspace  VariableName=TransportationChannel_15_Status  SaveFormat=Structure With Time  isMonitorOnly=off  isRecordIC=off
      settings: SourceProductName=SimEvents  SourceProductBaseCode=SE
  Timed to Event Signal : TimedToEventSignal
  TravelTime : Constant  Value=130.2958/30
  IN_Shipment_1 : PMIOPort  Side=Left
  OUT_Shipment_1 : PMIOPort  Port=2  Side=Right
  IN_Resource_1 : PMIOPort  Port=3  Side=Left
  OUT_Resource_1 : PMIOPort  Port=4  Side=Right
  IN_Shipment_2 : PMIOPort  Port=5  Side=Left
  OUT_Shipment_2 : PMIOPort  Port=6  Side=Right
  IN_Resource_2 : PMIOPort  Port=7  Side=Left
  OUT_Resource_2 : PMIOPort  Port=8  Side=Right
  tag scope: TransportationChannel_15_Status=global
  wires:
  Sum4/1 -> Mux/3
  Inbound_Process_2/1 -> Sum4/2
  Inbound_Process_1/1 -> Sum4/1
  Inbound_Process_2/2 -> Sum3/4
  Outbound_Process_2/1 -> Sum3/3
  Inbound_Process_1/2 -> Sum3/2
  Outbound_Process_1/1 -> Sum3/1
  Sum3/1 -> Mux/2
  Sum/1 -> Mux/1
  Mux/1 -> TC_Status/1, [TransportationChannel_15_Status]
  Inbound_Release_2/1 -> Sum2/2
  Outbound_Release_1/1 -> Sum2/1
  Sum2/1 -> Enabled Gate/1
  Inbound_Release_1/1 -> Sum1/1
  Outbound_Release_2/1 -> Sum1/2
  Sum1/1 -> Enabled Gate1/1
  Timed to Event Signal/1 -> Outbound_Process_2/1, Outbound_Process_1/1, Infinite Server1/1, Inbound_Process_2/1, Inbound_Process_1/1, Infinite Server/1
  TravelTime/1 -> Timed to Event Signal/1
  FIFO Queue/1 -> Sum/1
  FIFO Queue1/1 -> Sum/2
  connections:
  Inbound_Process_1/RConn1 -- OUT_Resource_1/RConn1
  Outbound_Process_1/RConn1 -- Inbound_Release_1/LConn1
  Inbound_Release_1/RConn1 -- Inbound_Process_1/LConn1
  Outbound_Release_1/RConn1 -- Outbound_Process_1/LConn1
  Inbound_Process_2/RConn1 -- OUT_Resource_2/RConn1
  Inbound_Release_2/RConn1 -- Inbound_Process_2/LConn1
  Outbound_Process_2/RConn1 -- Inbound_Release_2/LConn1
  Outbound_Release_2/RConn1 -- Outbound_Process_2/LConn1
  IN_Resource_2/RConn1 -- Outbound_Release_2/LConn1
  Infinite Server1/RConn1 -- OUT_Shipment_1/RConn1
  Enabled Gate/RConn1 -- Infinite Server1/LConn1
  Infinite Server/LConn1 -- Enabled Gate1/RConn1
  OUT_Shipment_2/RConn1 -- Infinite Server/RConn1
  IN_Resource_1/RConn1 -- Outbound_Release_1/LConn1
  IN_Shipment_2/RConn1 -- FIFO Queue1/LConn1
  IN_Shipment_1/RConn1 -- FIFO Queue/LConn1
  Enabled Gate1/LConn1 -- FIFO Queue1/RConn1
  FIFO Queue/RConn1 -- Enabled Gate/LConn1

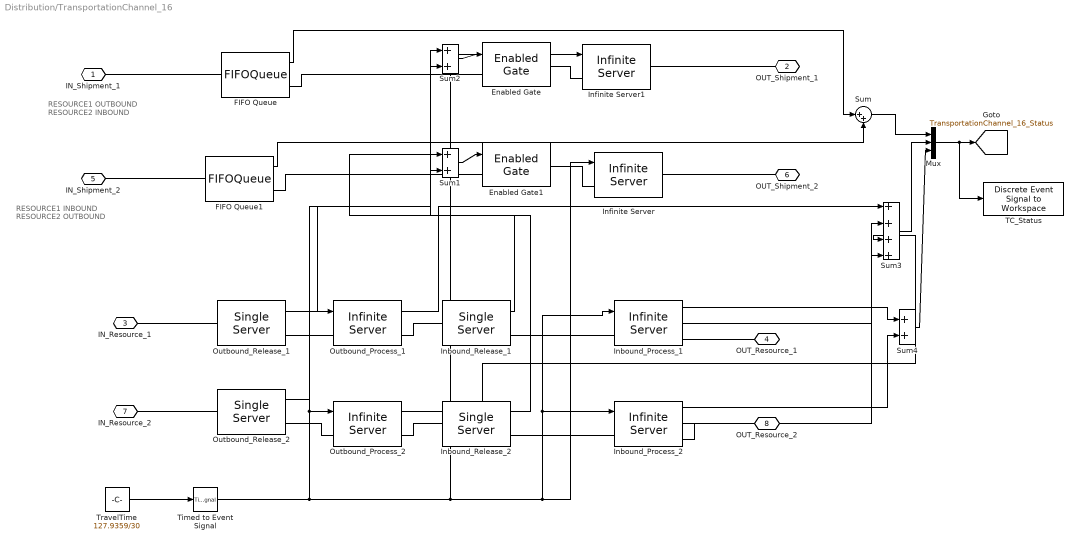
== system Distribution/TransportationChannel_16 ==
  note: RESOURCE1 OUTBOUND
      | RESOURCE2 INBOUND
  note: RESOURCE1 INBOUND
      | RESOURCE2 OUTBOUND
  Enabled Gate : EnabledGate
  Enabled Gate1 : EnabledGate
  FIFO Queue : FIFOQueue  Capacity=inf  StatNumberInBlock=on
      settings: OutputPortMap=o1
  FIFO Queue1 : FIFOQueue  Capacity=inf  StatNumberInBlock=on
      settings: OutputPortMap=o1
  Inbound_Process_1 : InfiniteServer  ServiceTimeFrom=Signal port t  ServiceTime=(76.7)/30  StatNumberDeparted=on  StatNumberInBlock=on
      settings: OutputPortMap=o0,o1
  Inbound_Process_2 : InfiniteServer  ServiceTimeFrom=Signal port t  ServiceTime=(76.7)/30  StatNumberDeparted=on  StatNumberInBlock=on
      settings: OutputPortMap=o0,o1
  Inbound_Release_1 : SingleServer  ServiceTime=0  StatNumberInBlock=on
      settings: OutputPortMap=o1
  Inbound_Release_2 : SingleServer  ServiceTime=0  StatNumberInBlock=on
      settings: OutputPortMap=o1
  Infinite Server : InfiniteServer  ServiceTimeFrom=Signal port t  ServiceTime=(76.7)/30
  Infinite Server1 : InfiniteServer  ServiceTimeFrom=Signal port t  ServiceTime=(76.7)/30
  Mux : Mux  Inputs=3
  Outbound_Process_1 : InfiniteServer  ServiceTimeFrom=Signal port t  ServiceTime=(76.7)/30  StatNumberInBlock=on
      settings: OutputPortMap=o1
  Outbound_Process_2 : InfiniteServer  ServiceTimeFrom=Signal port t  ServiceTime=(76.7)/30  StatNumberInBlock=on
      settings: OutputPortMap=o1
  Outbound_Release_1 : SingleServer  ServiceTime=0  StatNumberInBlock=on
      settings: OutputPortMap=o1
  Outbound_Release_2 : SingleServer  ServiceTime=0  StatNumberInBlock=on
      settings: OutputPortMap=o1
  Sum{,1..2,4} (4 alike) : Sum  Inputs=|++
  Sum3 : Sum  Inputs=|++++
  TC_Status : simeventslib/SimEvents Sinks/Discrete Event Signal to Workspace  VariableName=TransportationChannel_16_Status  SaveFormat=Structure With Time  isMonitorOnly=off  isRecordIC=off
      settings: SourceProductName=SimEvents  SourceProductBaseCode=SE
  Timed to Event Signal : TimedToEventSignal
  TravelTime : Constant  Value=127.9359/30
  IN_Shipment_1 : PMIOPort  Side=Left
  OUT_Shipment_1 : PMIOPort  Port=2  Side=Right
  IN_Resource_1 : PMIOPort  Port=3  Side=Left
  OUT_Resource_1 : PMIOPort  Port=4  Side=Right
  IN_Shipment_2 : PMIOPort  Port=5  Side=Left
  OUT_Shipment_2 : PMIOPort  Port=6  Side=Right
  IN_Resource_2 : PMIOPort  Port=7  Side=Left
  OUT_Resource_2 : PMIOPort  Port=8  Side=Right
  tag scope: TransportationChannel_16_Status=global
  wires:
  Sum4/1 -> Mux/3
  Inbound_Process_2/1 -> Sum4/2
  Inbound_Process_1/1 -> Sum4/1
  Inbound_Process_2/2 -> Sum3/4
  Outbound_Process_2/1 -> Sum3/3
  Inbound_Process_1/2 -> Sum3/2
  Outbound_Process_1/1 -> Sum3/1
  Sum3/1 -> Mux/2
  Sum/1 -> Mux/1
  Mux/1 -> TC_Status/1, [TransportationChannel_16_Status]
  Inbound_Release_2/1 -> Sum2/2
  Outbound_Release_1/1 -> Sum2/1
  Sum2/1 -> Enabled Gate/1
  Inbound_Release_1/1 -> Sum1/1
  Outbound_Release_2/1 -> Sum1/2
  Sum1/1 -> Enabled Gate1/1
  Timed to Event Signal/1 -> Outbound_Process_2/1, Outbound_Process_1/1, Infinite Server1/1, Inbound_Process_2/1, Inbound_Process_1/1, Infinite Server/1
  TravelTime/1 -> Timed to Event Signal/1
  FIFO Queue/1 -> Sum/1
  FIFO Queue1/1 -> Sum/2
  connections:
  Inbound_Process_1/RConn1 -- OUT_Resource_1/RConn1
  Outbound_Process_1/RConn1 -- Inbound_Release_1/LConn1
  Inbound_Release_1/RConn1 -- Inbound_Process_1/LConn1
  Outbound_Release_1/RConn1 -- Outbound_Process_1/LConn1
  Inbound_Process_2/RConn1 -- OUT_Resource_2/RConn1
  Inbound_Release_2/RConn1 -- Inbound_Process_2/LConn1
  Outbound_Process_2/RConn1 -- Inbound_Release_2/LConn1
  Outbound_Release_2/RConn1 -- Outbound_Process_2/LConn1
  IN_Resource_2/RConn1 -- Outbound_Release_2/LConn1
  Infinite Server1/RConn1 -- OUT_Shipment_1/RConn1
  Enabled Gate/RConn1 -- Infinite Server1/LConn1
  Infinite Server/LConn1 -- Enabled Gate1/RConn1
  OUT_Shipment_2/RConn1 -- Infinite Server/RConn1
  IN_Resource_1/RConn1 -- Outbound_Release_1/LConn1
  IN_Shipment_2/RConn1 -- FIFO Queue1/LConn1
  IN_Shipment_1/RConn1 -- FIFO Queue/LConn1
  Enabled Gate1/LConn1 -- FIFO Queue1/RConn1
  FIFO Queue/RConn1 -- Enabled Gate/LConn1

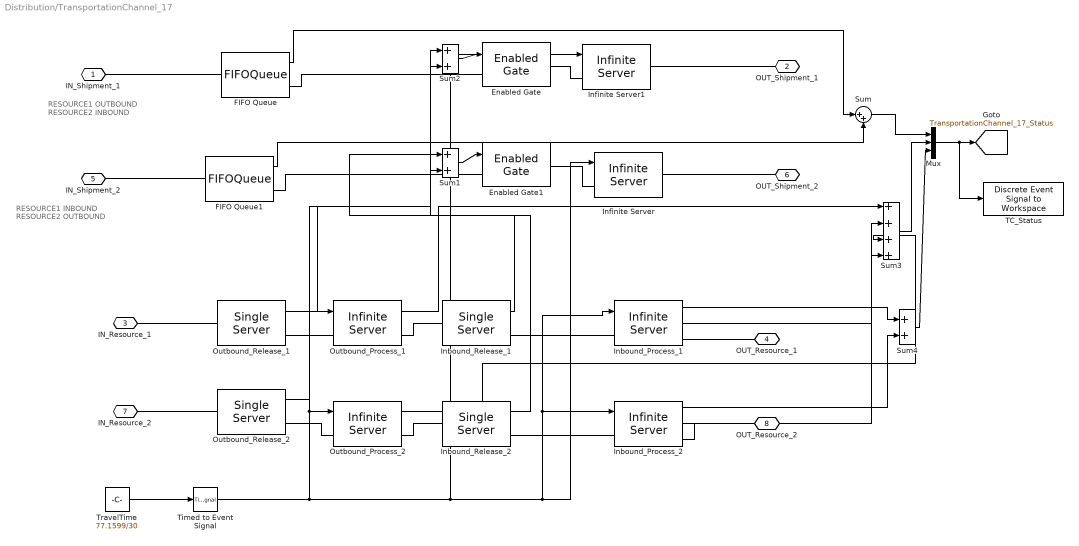
== system Distribution/TransportationChannel_17 ==
  note: RESOURCE1 OUTBOUND
      | RESOURCE2 INBOUND
  note: RESOURCE1 INBOUND
      | RESOURCE2 OUTBOUND
  Enabled Gate : EnabledGate
  Enabled Gate1 : EnabledGate
  FIFO Queue : FIFOQueue  Capacity=inf  StatNumberInBlock=on
      settings: OutputPortMap=o1
  FIFO Queue1 : FIFOQueue  Capacity=inf  StatNumberInBlock=on
      settings: OutputPortMap=o1
  Inbound_Process_1 : InfiniteServer  ServiceTimeFrom=Signal port t  ServiceTime=(76.7)/30  StatNumberDeparted=on  StatNumberInBlock=on
      settings: OutputPortMap=o0,o1
  Inbound_Process_2 : InfiniteServer  ServiceTimeFrom=Signal port t  ServiceTime=(76.7)/30  StatNumberDeparted=on  StatNumberInBlock=on
      settings: OutputPortMap=o0,o1
  Inbound_Release_1 : SingleServer  ServiceTime=0  StatNumberInBlock=on
      settings: OutputPortMap=o1
  Inbound_Release_2 : SingleServer  ServiceTime=0  StatNumberInBlock=on
      settings: OutputPortMap=o1
  Infinite Server : InfiniteServer  ServiceTimeFrom=Signal port t  ServiceTime=(76.7)/30
  Infinite Server1 : InfiniteServer  ServiceTimeFrom=Signal port t  ServiceTime=(76.7)/30
  Mux : Mux  Inputs=3
  Outbound_Process_1 : InfiniteServer  ServiceTimeFrom=Signal port t  ServiceTime=(76.7)/30  StatNumberInBlock=on
      settings: OutputPortMap=o1
  Outbound_Process_2 : InfiniteServer  ServiceTimeFrom=Signal port t  ServiceTime=(76.7)/30  StatNumberInBlock=on
      settings: OutputPortMap=o1
  Outbound_Release_1 : SingleServer  ServiceTime=0  StatNumberInBlock=on
      settings: OutputPortMap=o1
  Outbound_Release_2 : SingleServer  ServiceTime=0  StatNumberInBlock=on
      settings: OutputPortMap=o1
  Sum{,1..2,4} (4 alike) : Sum  Inputs=|++
  Sum3 : Sum  Inputs=|++++
  TC_Status : simeventslib/SimEvents Sinks/Discrete Event Signal to Workspace  VariableName=TransportationChannel_17_Status  SaveFormat=Structure With Time  isMonitorOnly=off  isRecordIC=off
      settings: SourceProductName=SimEvents  SourceProductBaseCode=SE
  Timed to Event Signal : TimedToEventSignal
  TravelTime : Constant  Value=77.1599/30
  IN_Shipment_1 : PMIOPort  Side=Left
  OUT_Shipment_1 : PMIOPort  Port=2  Side=Right
  IN_Resource_1 : PMIOPort  Port=3  Side=Left
  OUT_Resource_1 : PMIOPort  Port=4  Side=Right
  IN_Shipment_2 : PMIOPort  Port=5  Side=Left
  OUT_Shipment_2 : PMIOPort  Port=6  Side=Right
  IN_Resource_2 : PMIOPort  Port=7  Side=Left
  OUT_Resource_2 : PMIOPort  Port=8  Side=Right
  tag scope: TransportationChannel_17_Status=global
  wires:
  Sum4/1 -> Mux/3
  Inbound_Process_2/1 -> Sum4/2
  Inbound_Process_1/1 -> Sum4/1
  Inbound_Process_2/2 -> Sum3/4
  Outbound_Process_2/1 -> Sum3/3
  Inbound_Process_1/2 -> Sum3/2
  Outbound_Process_1/1 -> Sum3/1
  Sum3/1 -> Mux/2
  Sum/1 -> Mux/1
  Mux/1 -> TC_Status/1, [TransportationChannel_17_Status]
  Inbound_Release_2/1 -> Sum2/2
  Outbound_Release_1/1 -> Sum2/1
  Sum2/1 -> Enabled Gate/1
  Inbound_Release_1/1 -> Sum1/1
  Outbound_Release_2/1 -> Sum1/2
  Sum1/1 -> Enabled Gate1/1
  Timed to Event Signal/1 -> Outbound_Process_2/1, Outbound_Process_1/1, Infinite Server1/1, Inbound_Process_2/1, Inbound_Process_1/1, Infinite Server/1
  TravelTime/1 -> Timed to Event Signal/1
  FIFO Queue/1 -> Sum/1
  FIFO Queue1/1 -> Sum/2
  connections:
  Inbound_Process_1/RConn1 -- OUT_Resource_1/RConn1
  Outbound_Process_1/RConn1 -- Inbound_Release_1/LConn1
  Inbound_Release_1/RConn1 -- Inbound_Process_1/LConn1
  Outbound_Release_1/RConn1 -- Outbound_Process_1/LConn1
  Inbound_Process_2/RConn1 -- OUT_Resource_2/RConn1
  Inbound_Release_2/RConn1 -- Inbound_Process_2/LConn1
  Outbound_Process_2/RConn1 -- Inbound_Release_2/LConn1
  Outbound_Release_2/RConn1 -- Outbound_Process_2/LConn1
  IN_Resource_2/RConn1 -- Outbound_Release_2/LConn1
  Infinite Server1/RConn1 -- OUT_Shipment_1/RConn1
  Enabled Gate/RConn1 -- Infinite Server1/LConn1
  Infinite Server/LConn1 -- Enabled Gate1/RConn1
  OUT_Shipment_2/RConn1 -- Infinite Server/RConn1
  IN_Resource_1/RConn1 -- Outbound_Release_1/LConn1
  IN_Shipment_2/RConn1 -- FIFO Queue1/LConn1
  IN_Shipment_1/RConn1 -- FIFO Queue/LConn1
  Enabled Gate1/LConn1 -- FIFO Queue1/RConn1
  FIFO Queue/RConn1 -- Enabled Gate/LConn1
